simulink model "ev"  (R2019a)
settings: Solver=FixedStepAuto  StartTime=0  StopTime=30  RelTol=1e-3  AbsTol=1e-3
PreLoadFcn:
  | % Simulation parameters
  | dt = 0.01;
  | 
  | % Battery cell parameters
  | ssc_lithium_cell_1RC_ini
  | 
  | % Motor parameters
  | max_torque = 220;
  | max_power = 50e3;
  | 
  | % Vehicle parameters
  | vehicle_mass = 1000;
  | wheel_radius = 0.25;
  | area = 5;
  | drag_coefficient = 0.25;
  | air_density = 1.225;
  | gravity = 9.81;
  | rolling_res_ratio = 0.015;
  | 
  | % Differential drive parameters
  | gear_ratio = 6;
  | 
  | % Simplified braking system parameters
  | force_max_pedal = 500;
  | braking_torque_to_pedal_force_ratio = -4;
  | 
  | % Vehicle controller parameters
  | hill_hold_max_speed = 0.5;
  | 
  | % Water properties for cooling circuit
  | load WaterProperties
undefined symbols (not defined in the file): C1_LUT, Capacity_LUT, cell_Cp_heat, cell_mass, DiscIntNeverNeededParam, Em_LUT, Qe_init, R0_LUT, R1_LUT, sigbuilder_block, SOC_LUT, T_init, Temperature_LUT
libraries: fl_lib x57, fl_ps_legacy_lib x36, nesl_utility x13, LiBatteryElements_lib x4, autolibshared x3, ee_lib x2, simulink x2, simulink_extras x1
(part 2 of 2)

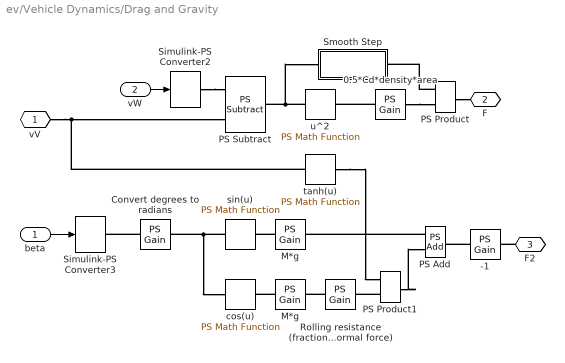
== system ev/Vehicle Dynamics/Drag and Gravity ==
  beta : Inport
  vW : Inport  Port=2
  " M*g " : fl_ps_legacy_lib/Legacy Physical Signals/Functions/PS Gain  gain=vehicle_mass*gravity
      settings: SourceProductName=Foundation Library
  -1 : fl_ps_legacy_lib/Legacy Physical Signals/Functions/PS Gain  gain=-1
      settings: SourceProductName=Foundation Library
  0.5*Cd*density*area : fl_ps_legacy_lib/Legacy Physical Signals/Functions/PS Gain  gain=0.5*drag_coefficient*air_density*area
      settings: SourceProductName=Foundation Library
  "Convert degrees to radians " : fl_ps_legacy_lib/Legacy Physical Signals/Functions/PS Gain  gain=pi/180
      settings: SourceProductName=Foundation Library
  M*g : fl_ps_legacy_lib/Legacy Physical Signals/Functions/PS Gain  gain=vehicle_mass*gravity
      settings: SourceProductName=Foundation Library
  PS Add : fl_ps_legacy_lib/Legacy Physical Signals/Functions/PS Add
      settings: SourceProductName=Foundation Library
  PS Product : fl_ps_legacy_lib/Legacy Physical Signals/Functions/PS Product
      settings: SourceProductName=Foundation Library
  PS Product1 : fl_ps_legacy_lib/Legacy Physical Signals/Functions/PS Product
      settings: SourceProductName=Foundation Library
  PS Subtract : fl_ps_legacy_lib/Legacy Physical Signals/Functions/PS Subtract
      settings: SourceProductName=Foundation Library
  "Rolling resistance (fraction of normal force) " : fl_ps_legacy_lib/Legacy Physical Signals/Functions/PS Gain  gain=rolling_res_ratio
      settings: SourceProductName=Foundation Library
  Simulink-PS Converter2 : nesl_utility/Simulink-PS Converter  PhysicalDomain=network_engine_domain  SubClassName=ps_input  LeftPortType=input  RightPortType=output  PseudoPeriodic=off  Frequencies=[]  NoiseDistribution=none  NoiseParameters=[]  Unit=N*m  AffineConversion=off  FilteringAndDerivatives=zero  SimscapeFilterOrder=1  InputFilterTimeConstant=0.001  UdotUserProvided=1
  Simulink-PS Converter3 : nesl_utility/Simulink-PS Converter  PhysicalDomain=network_engine_domain  SubClassName=ps_input  LeftPortType=input  RightPortType=output  PseudoPeriodic=off  Frequencies=[]  NoiseDistribution=none  NoiseParameters=[]  Unit=N*m  AffineConversion=off  FilteringAndDerivatives=zero  SimscapeFilterOrder=1  InputFilterTimeConstant=0.001  UdotUserProvided=1
  Smooth Step : Subsystem
  cos(u) : fl_ps_legacy_lib/Legacy Physical Signals/Functions/PS Math Function  fcn_choice=2
      settings: SourceProductName=Foundation Library
  sin(u) : fl_ps_legacy_lib/Legacy Physical Signals/Functions/PS Math Function  fcn_choice=1
      settings: SourceProductName=Foundation Library
  tanh(u) : fl_ps_legacy_lib/Legacy Physical Signals/Functions/PS Math Function  fcn_choice=10
      settings: SourceProductName=Foundation Library
  u^2 : fl_ps_legacy_lib/Legacy Physical Signals/Functions/PS Math Function  fcn_choice=7
      settings: SourceProductName=Foundation Library
  vV : PMIOPort  Side=Left
  F : PMIOPort  Port=2  Side=Left
  F2 : PMIOPort  Port=3  Side=Left
  wires:
  vW/1 -> Simulink-PS Converter2/1
  beta/1 -> Simulink-PS Converter3/1
  connections:
  vV/RConn1 -- tanh(u)/LConn1 -- PS Subtract/LConn1
  Simulink-PS Converter2/RConn1 -- PS Subtract/LConn2
  u^2/LConn1 -- Smooth Step/LConn1 -- PS Subtract/RConn1
  0.5*Cd*density*area/LConn1 -- u^2/RConn1
  0.5*Cd*density*area/RConn1 -- PS Product/LConn2
  PS Product/RConn1 -- F/RConn1
  PS Product/LConn1 -- Smooth Step/RConn1
  "Convert degrees to radians "/LConn1 -- Simulink-PS Converter3/RConn1
  sin(u)/LConn1 -- "Convert degrees to radians "/RConn1 -- cos(u)/LConn1
  M*g/LConn1 -- sin(u)/RConn1
  " M*g "/LConn1 -- cos(u)/RConn1
  "Rolling resistance (fraction of normal force) "/LConn1 -- " M*g "/RConn1
  PS Product1/LConn2 -- "Rolling resistance (fraction of normal force) "/RConn1
  PS Add/LConn1 -- M*g/RConn1
  PS Product1/RConn1 -- PS Add/LConn2
  -1/LConn1 -- PS Add/RConn1
  F2/RConn1 -- -1/RConn1
  tanh(u)/RConn1 -- PS Product1/LConn1

== system ev/Vehicle Dynamics/Sensing Speed ==
  MTRef : fl_lib/Mechanical/Translational Elements/Mechanical Translational Reference
      settings: SourceProductName=Foundation Library
  Motion Sensor : fl_lib/Mechanical/Mechanical Sensors/Ideal Translational Motion Sensor  offset=0 m
      settings: SourceProductName=Foundation Library
  PS-Simulink Converter3 : nesl_utility/PS-Simulink Converter  PhysicalDomain=network_engine_domain  SubClassName=ps_output  LeftPortType=input  RightPortType=output  PseudoPeriodic=off  Frequencies=[]  Unit=mph  AffineConversion=off
  R : PMIOPort  Side=Left
  w : PMIOPort  Port=2  Side=Right
  tag scope: vSpd=global
  wires:
  PS-Simulink Converter3/1 -> [vSpd]  "Vehicle Speed"
  connections:
  R/RConn1 -- Motion Sensor/LConn1
  MTRef/LConn1 -- Motion Sensor/RConn1
  Motion Sensor/RConn2 -- PS-Simulink Converter3/LConn1 -- w/RConn1

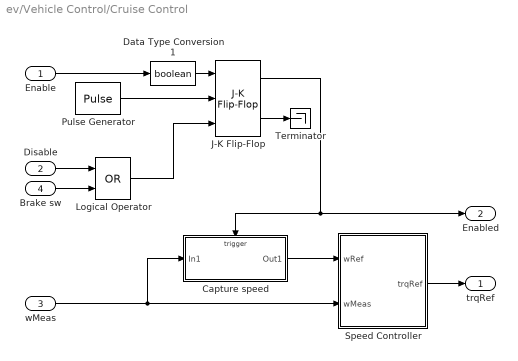
== system ev/Vehicle Control/Cruise Control ==
  Enable : Inport
  Disable : Inport  Port=2
  wMeas : Inport  Port=3
  Brake sw : Inport  Port=4
  Capture speed : Subsystem  TreatAsAtomicUnit=on
  Data Type Conversion1 : DataTypeConversion  OutDataTypeStr=boolean
  J-K Flip-Flop : simulink_extras/Flip Flops/J-K Flip-Flop  initial_condition=0
      settings: SourceProductName=Simulink Extras
  Logical Operator : Logic  Operator=OR  AllPortsSameDT=off  OutDataTypeStr=boolean
  Pulse Generator : DiscretePulseGenerator  Period=10  PulseWidth=5  SampleTime=0.01
  Speed Controller : Subsystem  mask(P+I motor speed controller){Kp=100, Ki=100, trqMax=max_torque, ts=dt}
      mask prompts: Kp "Proportional gain (Nm/(rad/s))"; Ki "Integral gain (Nm/rad)"; trqMax "Maximum torque demand"; ts "Sample time"
      mask help: Inputs wRef and wMeas are the demanded rotor speed and measured rotor speed in rad/s. The controller output is a torque demand in Nm.
  Terminator : Terminator
  trqRef : Outport
  Enabled : Outport  Port=2
  wires:
  Enable/1 -> Data Type Conversion1/1
  Pulse Generator/1 -> J-K Flip-Flop/2
  Disable/1 -> Logical Operator/1
  Speed Controller/1(trqRef) -> trqRef/1
  Brake sw/1 -> Logical Operator/2
  wMeas/1 -> Capture speed/1(In1), Speed Controller/2(wMeas)
  Logical Operator/1 -> J-K Flip-Flop/3
  J-K Flip-Flop/1 -> Enabled/1, Capture speed/Trigger
  Data Type Conversion1/1 -> J-K Flip-Flop/1
  J-K Flip-Flop/2 -> Terminator/1
  Capture speed/1(Out1) -> Speed Controller/1(wRef)

== system ev/Vehicle Control/Feedforward term for regenerative braking on downhill ==
  Inclin. : Inport
  " M " : Gain  Gain=vehicle_mass
  1/ratio : Gain  Gain=1/gear_ratio
  Wheel radius : Gain  Gain=wheel_radius
  Feedfwd trq : Outport
  wires:
  Inclin./1 -> " M "/1
  " M "/1 -> Wheel radius/1
  Wheel radius/1 -> 1/ratio/1  "Wheel torque"
  1/ratio/1 -> Feedfwd trq/1  "Motor torque"

== system ev/Vehicle Control/Max Power ==
  Vspd : Inport
  Abs : Abs
  Constant : Constant
  Math Function : Math  Operator=reciprocal  SaturateOnIntegerOverflow=on
  Prevent divide by zero : Switch  Criteria=u2 > Threshold  Threshold=1
  max_power : Gain  Gain=max_power
  Max Power : Outport
  wires:
  Prevent divide by zero/1 -> Math Function/1
  Constant/1 -> Prevent divide by zero/3
  Abs/1 -> Prevent divide by zero/2, Prevent divide by zero/1
  Math Function/1 -> max_power/1
  max_power/1 -> Max Power/1
  Vspd/1 -> Abs/1

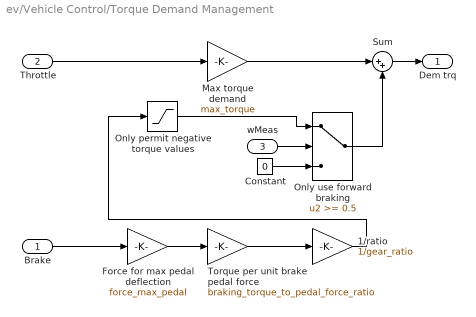
== system ev/Vehicle Control/Torque Demand Management ==
  Brake : Inport
  Throttle : Inport  Port=2
  wMeas : Inport  Port=3
  1/ratio : Gain  Gain=1/gear_ratio
  Constant : Constant  Value=0  SampleTime=dt
  Force for max pedal deflection : Gain  Gain=force_max_pedal
  Max torque demand : Gain  Gain=max_torque
  Only permit negative torque values : Saturate  UpperLimit=-10  LowerLimit=-max_torque
  Only use forward braking : Switch  Threshold=0.5  InputSameDT=on
  Sum : Sum  Inputs=|++
  Torque per unit brake pedal force : Gain  Gain=braking_torque_to_pedal_force_ratio
  Dem trq : Outport
  wires:
  Max torque demand/1 -> Sum/1
  Brake/1 -> Force for max pedal deflection/1
  Sum/1 -> Dem trq/1
  Throttle/1 -> Max torque demand/1
  Torque per unit brake pedal force/1 -> 1/ratio/1
  1/ratio/1 -> Only permit negative torque values/1
  Force for max pedal deflection/1 -> Torque per unit brake pedal force/1
  wMeas/1 -> Only use forward braking/2
  Only use forward braking/1 -> Sum/2
  Constant/1 -> Only use forward braking/3
  Only permit negative torque values/1 -> Only use forward braking/1

== system ev/Cooling System/Heat Exch. Characteristic/Characteristic ==
  PS Product : fl_ps_legacy_lib/Legacy Physical Signals/Functions/PS Product
      settings: SourceProductName=Foundation Library
  PS Subtract : fl_ps_legacy_lib/Legacy Physical Signals/Functions/PS Subtract
      settings: SourceProductName=Foundation Library
  Specific dissipation (J/s/K) per unit mass flow rate : fl_ps_legacy_lib/Legacy Physical Signals/Functions/PS Gain  gain=100
      settings: SourceProductName=Foundation Library
  M : PMIOPort  Side=Right
  T in : PMIOPort  Port=2  Side=Right
  T Env : PMIOPort  Port=3  Side=Right
  Q : PMIOPort  Port=4  Side=Left
  connections:
  T Env/RConn1 -- PS Subtract/LConn1
  PS Product/RConn1 -- Q/RConn1
  PS Subtract/RConn1 -- PS Product/LConn1
  T in/RConn1 -- PS Subtract/LConn2
  M/RConn1 -- Specific dissipation (J/s/K) per unit mass flow rate/LConn1
  PS Product/LConn2 -- Specific dissipation (J/s/K) per unit mass flow rate/RConn1

== system ev/PMSM Drive/Heat Exch. Characteristic/Characteristic ==
  PS Product : fl_ps_legacy_lib/Legacy Physical Signals/Functions/PS Product
      settings: SourceProductName=Foundation Library
  PS Subtract : fl_ps_legacy_lib/Legacy Physical Signals/Functions/PS Subtract
      settings: SourceProductName=Foundation Library
  Specific dissipation (J/s/K) : fl_ps_legacy_lib/Legacy Physical Signals/Lookup Tables/PS Lookup Table (1D)  x="[0 0.2 0.4  0.7  1 1.2  1.4  2.5 ]"  f=100 * [0 0.5 0.75 0.92 1 1.02 1.03 1.04]  interp_method=1  extrap_method=1
      settings: SourceProductName=Foundation Library
  Specific dissipation (J/s/K) per unit mass flow rate : fl_ps_legacy_lib/Legacy Physical Signals/Functions/PS Gain  gain=100
      settings: SourceProductName=Foundation Library
  Mass Flow : PMIOPort  Side=Left
  Temp Inlet : PMIOPort  Port=2  Side=Left
  Temp Motor : PMIOPort  Port=3  Side=Left
  Q : PMIOPort  Port=4  Side=Right
  connections:
  PS Subtract/RConn1 -- PS Product/LConn1
  Specific dissipation (J/s/K)/RConn1 -- PS Product/LConn2
  Temp Motor/RConn1 -- PS Subtract/LConn1
  PS Subtract/LConn2 -- Temp Inlet/RConn1
  PS Product/RConn1 -- Q/RConn1
  Mass Flow/RConn1 -- Specific dissipation (J/s/K) per unit mass flow rate/LConn1
  Specific dissipation (J/s/K) per unit mass flow rate/RConn1 -- Specific dissipation (J/s/K)/LConn1

== system ev/Vehicle Dynamics/Brake Torque/Smooth Sign ==
  1 : fl_lib/Physical Signals/Sources/PS Constant  constant=1
      settings: SourceProductName=Foundation Library
  2 : fl_ps_legacy_lib/Legacy Physical Signals/Functions/PS Gain  gain=2
      settings: SourceProductName=Foundation Library
  exp(2x) : fl_ps_legacy_lib/Legacy Physical Signals/Functions/PS Math Function  fcn_choice=3
      settings: SourceProductName=Foundation Library
  exp(2x)+1 : fl_ps_legacy_lib/Legacy Physical Signals/Functions/PS Add
      settings: SourceProductName=Foundation Library
  exp(2x)-1 : fl_ps_legacy_lib/Legacy Physical Signals/Functions/PS Subtract
      settings: SourceProductName=Foundation Library
  tanh(x) : fl_ps_legacy_lib/Legacy Physical Signals/Functions/PS Divide
      settings: SourceProductName=Foundation Library
  x : PMIOPort  Side=Left
  y : PMIOPort  Port=2  Side=Right
  connections:
  y/RConn1 -- tanh(x)/RConn1
  x/RConn1 -- 2/LConn1
  exp(2x)-1/RConn1 -- tanh(x)/LConn1
  exp(2x)+1/RConn1 -- tanh(x)/LConn2
  exp(2x)+1/LConn2 -- exp(2x)-1/LConn1 -- exp(2x)/RConn1
  2/RConn1 -- exp(2x)/LConn1
  exp(2x)-1/LConn2 -- exp(2x)+1/LConn1 -- 1/RConn1

== system ev/Vehicle Dynamics/Drag and Gravity/Smooth Step ==
  1 : fl_lib/Physical Signals/Sources/PS Constant  constant=1
      settings: SourceProductName=Foundation Library
  2 : fl_ps_legacy_lib/Legacy Physical Signals/Functions/PS Gain  gain=2
      settings: SourceProductName=Foundation Library
  exp(2x) : fl_ps_legacy_lib/Legacy Physical Signals/Functions/PS Math Function  fcn_choice=3
      settings: SourceProductName=Foundation Library
  exp(2x)+1 : fl_ps_legacy_lib/Legacy Physical Signals/Functions/PS Add
      settings: SourceProductName=Foundation Library
  exp(2x)-1 : fl_ps_legacy_lib/Legacy Physical Signals/Functions/PS Subtract
      settings: SourceProductName=Foundation Library
  tanh(x) : fl_ps_legacy_lib/Legacy Physical Signals/Functions/PS Divide
      settings: SourceProductName=Foundation Library
  x : PMIOPort  Side=Left
  y : PMIOPort  Port=2  Side=Right
  connections:
  y/RConn1 -- tanh(x)/RConn1
  x/RConn1 -- 2/LConn1
  exp(2x)-1/RConn1 -- tanh(x)/LConn1
  exp(2x)+1/RConn1 -- tanh(x)/LConn2
  exp(2x)+1/LConn2 -- exp(2x)-1/LConn1 -- exp(2x)/RConn1
  2/RConn1 -- exp(2x)/LConn1
  exp(2x)-1/LConn2 -- exp(2x)+1/LConn1 -- 1/RConn1

== system ev/Vehicle Control/Cruise Control/Capture speed ==
  In1 : Inport
  Trigger : TriggerPort  VariantControl=Variant
  Out1 : Outport
  wires:
  In1/1 -> Out1/1

== system ev/Vehicle Control/Cruise Control/Speed Controller ==
  wRef : Inport
  wMeas : Inport  Port=2
  Add : Sum  Inputs=|+-
  Add1 : Sum
  Discrete-Time Integrator : DiscreteIntegrator  gainval=Ki  SampleTime=ts  LimitOutput=on  UpperSaturationLimit=trqMax  LowerSaturationLimit=-trqMax  ICPrevOutput=DiscIntNeverNeededParam  ICPrevScaledInput=DiscIntNeverNeededParam
  Kp : Gain  Gain=Kp
  trqRef : Outport
  wires:
  wRef/1 -> Add/1
  Kp/1 -> Add1/1
  Discrete-Time Integrator/1 -> Add1/2
  wMeas/1 -> Add/2
  Add1/1 -> trqRef/1
  Add/1 -> Kp/1, Discrete-Time Integrator/1
